simulink model "LyapunovTeste"  (R2016a)
settings: Solver=ode23t  StartTime=0.0  StopTime=1.5  FixedStep=t_PWM/10  MaxStep=2e-6  RelTol=2e-4
values from neighbouring files (symbols this model uses):
  C1 = t_PWM * (N*Impp)*0.1/ (8 * (N*Vmpp)*0.0001)    [SolarPanelModel.m]
  k_v = 1/ (t_PWM*2500)    (= 20)    [SolarPanelModel.m]
  k_vc = 1/ (t_PWM*250)    (= 200)    [SolarPanelModel.m]
  ki = max(double(Ski))    [SolarPanelModel.m]
  N = 3    [SolarPanelModel.m]
  Rs = sol(3)    [SolarPanelModel.m]
  t_PWM = 20e-6    (= 2e-05)    [SolarPanelModel.m]
  Voc = Vocr + miu_Voc*(Tc - Tr) + m*Vt*log(G/Gr)    [SolarPanelModel.m]
libraries: powerlib x8, powerlib_extras x1
settings Model: Creator=frede  LastModifiedBy=frede
settings DataIOCC: LimitDataPoints=on  SaveFormat=Array
settings HardwareCC: ProdBitPerPointer=32  ProdLargestAtomicFloat=None  ProdIntDivRoundTo=Undefined  ProdEndianess=Unspecified  ProdWordSize=32  ProdHWDeviceType=32-bit Generic
settings ModelReferenceCC: PropagateSignalLabelsOutOfModel=off
settings ConfigComp: CovModelRefEnable=Off

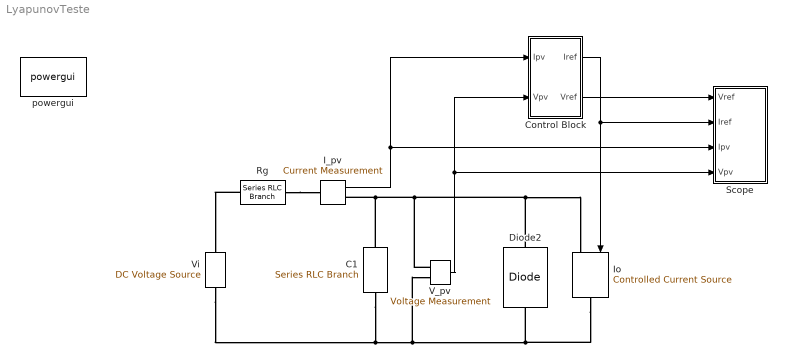
== system LyapunovTeste ==
  C1 : powerlib/Elements/Series RLC Branch  LConnTagsString=__new0  RConnTagsString=__new0  BranchType=C  Resistance=Rs  Inductance=1e-3  SetiL0=off  InitialCurrent=0  Capacitance=C1  Setx0=off  InitialVoltage=0  Measurements=None
  Control Block : Subsystem
  Diode2 : powerlib/Power Electronics/Diode  Ron=0.001  Lon=0  Vf=0.001  IC=0  UseSnubber=off  Rs=500  Cs=2e-9  Measurements=off
  I_pv : powerlib/Measurements/Current Measurement  PhasorSimulation=off  OutputType=Complex  PSBequivalent=0
  Io : powerlib/Electrical Sources/Controlled Current Source  Initialize=on  Source_Type=AC  Amplitude=0  Phase=0  Frequency=0  Measurements=None
  Rg : powerlib/Elements/Series RLC Branch  LConnTagsString=__new0  RConnTagsString=__new0  BranchType=R  Resistance=20  Inductance=1e-3  SetiL0=off  InitialCurrent=0  Capacitance=1e-6  Setx0=off  InitialVoltage=0  Measurements=None
  Scope : Subsystem
  V_pv : powerlib/Measurements/Voltage Measurement  PhasorSimulation=off  OutputType=Complex  PSBequivalent=0
  Vi : powerlib/Electrical Sources/DC Voltage Source  Amplitude=40  Measurements=None
  powergui : powerlib/powergui  Priority=1  SimulationMode=Discrete  SolverType=Tustin/Backward Euler (TBE)  SampleTime=t_PWM/10  frequency=60  SPID=off  DisableSnubberDevices=off  DisableRonSwitches=off  DisableVfSwitches=off  SwTol=0  DisplayEquations=off  Interpol=off  ExternalGateDelay=off  methode=off  Ts=10  FunctionMessages=off  echomessages=off  HookPort=off  EnableUseOfTLC=off  x0status=blocks  frequencyindice=0  Pbase=100e6  ErrMax=1e-4  Iterations=50  UnitsV=kV  UnitsW=MW  buscounter=0  RestoreLinks=warning  ResistiveCurrentMeasurement=off  Frange=[0:2:500]  Ylog=off  Xlog=on  ShowGrid=off  save=off  variable=ZData  structure=0  ZoomFFT=off  StartTime=0.0  cycles=1  DisplayStyle=1  fundamental=60  FreqAxis=off  MaxFrequency=1000  frequencyindicesteady=1  RmsSteady=1  display=off
  wires:
  Control Block/1(Iref) -> Scope/2(Iref), Io/1
  V_pv/1 -> Control Block/2(Vpv), Scope/4(Vpv)
  I_pv/1 -> Control Block/1(Ipv), Scope/3(Ipv)
  Control Block/2(Vref) -> Scope/1(Vref)
  connections:
  Diode2/RConn1 -- V_pv/LConn1 -- C1/LConn1 -- I_pv/RConn1 -- Io/LConn1
  Vi/LConn1 -- C1/RConn1 -- Io/RConn1 -- Diode2/LConn1 -- V_pv/LConn2
  Rg/RConn1 -- I_pv/LConn1
  Rg/LConn1 -- Vi/RConn1

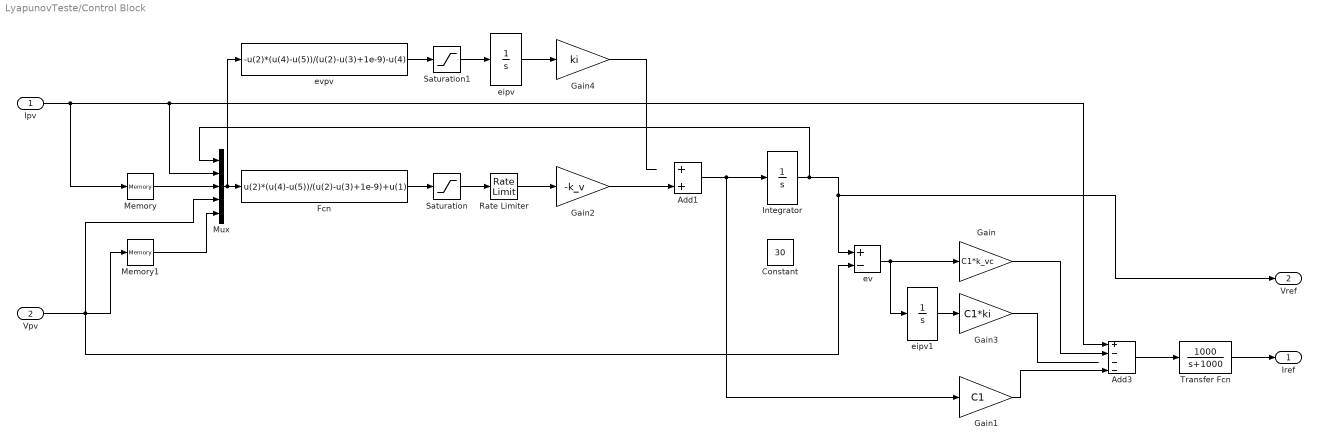
== system LyapunovTeste/Control Block ==
  Ipv : Inport
  Vpv : Inport  Port=2
  Add1 : Sum
  Add3 : Sum  Inputs=+---
  Constant : Constant  Value=30
  Fcn : Fcn  Expr=u(2)*(u(4)-u(5))/(u(2)-u(3)+1e-9)+u(1)
  Gain : Gain  Gain=C1*k_vc
  Gain1 : Gain  Gain=C1
  Gain2 : Gain  Gain=-k_v
  Gain3 : Gain  Gain=C1*ki
  Gain4 : Gain  Gain=ki
  Integrator : Integrator  InitialCondition=19  LimitOutput=on  UpperSaturationLimit=40  LowerSaturationLimit=0
  Memory : Memory
  Memory1 : Memory
  Mux : Mux  Inputs=5
  Rate Limiter : RateLimiter  RisingSlewLimit=1e6  FallingSlewLimit=-1e6  SampleTimeMode=inherited
  Saturation : Saturate  UpperLimit=140/k_v  LowerLimit=-Voc*N/k_v
  Saturation1 : Saturate  UpperLimit=Voc  LowerLimit=-Voc
  Transfer Fcn : TransferFcn  Numerator=[1000]  Denominator=[1 1000]
  eipv : Integrator  UpperSaturationLimit=Voc*N  LowerSaturationLimit=0
  eipv1 : Integrator  UpperSaturationLimit=Voc*N  LowerSaturationLimit=0
  ev : Sum  Inputs=+-
  evpv : Fcn  Expr=-u(2)*(u(4)-u(5))/(u(2)-u(3)+1e-9)-u(4)
  Iref : Outport
  Vref : Outport  Port=2
  wires:
  Add3/1 -> Transfer Fcn/1
  ev/1 -> eipv1/1, Gain/1
  Gain/1 -> Add3/2
  Gain1/1 -> Add3/4
  Add1/1 -> Gain1/1, Integrator/1
  Ipv/1 -> Mux/2, Add3/1, Memory/1
  Memory/1 -> Mux/3
  Memory1/1 -> Mux/5
  Vpv/1 -> ev/2, Memory1/1, Mux/4
  Fcn/1 -> Saturation/1
  Saturation/1 -> Rate Limiter/1
  Integrator/1 -> Vref/1, ev/1, Mux/1
  eipv1/1 -> Gain3/1
  Gain3/1 -> ?
  Gain2/1 -> Add1/2
  Mux/1 -> evpv/1, Fcn/1
  Rate Limiter/1 -> Gain2/1
  Saturation1/1 -> eipv/1
  eipv/1 -> Gain4/1
  Gain4/1 -> ?
  evpv/1 -> Saturation1/1
  Transfer Fcn/1 -> Iref/1

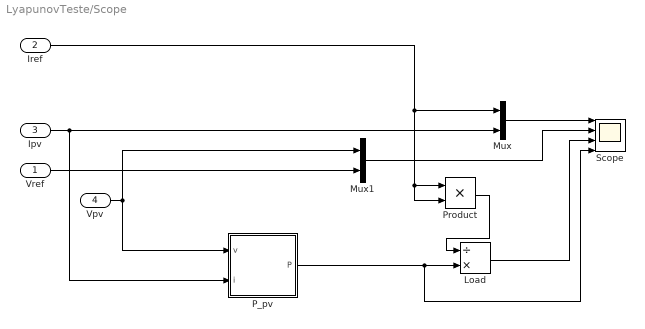
== system LyapunovTeste/Scope ==
  Vref : Inport
  Iref : Inport  Port=2
  Ipv : Inport  Port=3
  Vpv : Inport  Port=4
  Load : Product  Inputs=/*
  Mux : Mux  Inputs=2
  Mux1 : Mux  Inputs=2
  P_pv : Subsystem
  Product : Product  Inputs=**
  Scope : Scope  NumInputPorts=4
  wires:
  Mux/1 -> Scope/1
  P_pv/1(P) -> Scope/4, Load/2
  Mux1/1 -> Scope/2
  Ipv/1 -> Mux/2, P_pv/2(i)
  Vpv/1 -> Mux1/1, P_pv/1(v)
  Vref/1 -> Mux1/2
  Iref/1 -> Mux/1, Product/2, Product/1
  Load/1 -> Scope/3
  Product/1 -> Load/1

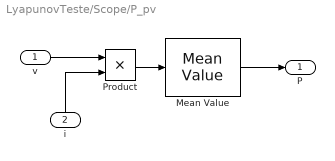
== system LyapunovTeste/Scope/P_pv ==
  v : Inport
  i : Inport  Port=2
  Mean Value : powerlib_extras/Measurements/Mean Value  Period=1/100
  Product : Product
  P : Outport
  wires:
  Mean Value/1 -> P/1
  Product/1 -> Mean Value/1
  v/1 -> Product/1
  i/1 -> Product/2
